simulink model "SELMOTOR_PELICAN_2025"  (R2025b)
settings: Solver=VariableStepAuto  StartTime=0.0  StopTime=5  RelTol=1e-3
settings Model: Creator=juanduque  LastModifiedBy=alvaro
settings SolverCC: AlgebraicLoopSolver=TrustRegion
settings DataIOCC: ReturnWorkspaceOutputs=off
settings OptimizationCC: ReuseModelBlockBuffer=off
settings DebuggingCC: UnconnectedInputMsg=warning  UnconnectedOutputMsg=warning  UnconnectedLineMsg=warning  ArithmeticOperatorsInVariantConditions=warning
settings ModelReferenceCC: EnableRefExpFcnMdlSchedulingChecks=on
settings SFSimCC: SimUseLocalCustomCode=off  CustomCodeUndefinedFunction=UseInterfaceOnly
settings RTWCC: RTWUseLocalCustomCode=off  GPUComputeCapability=3.5
settings CodeAppCC: StateflowObjectComments=on

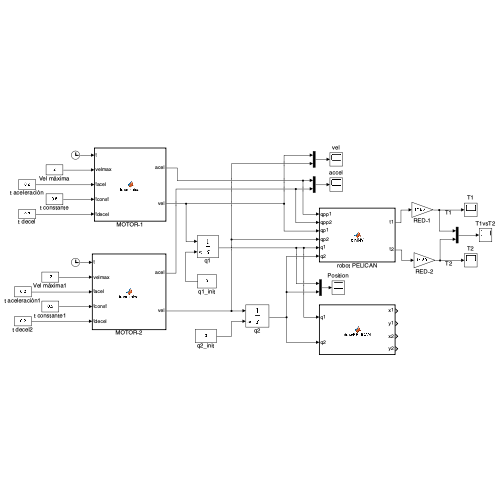
[thumbnail: Simulink's stored preview of the top-level diagram]
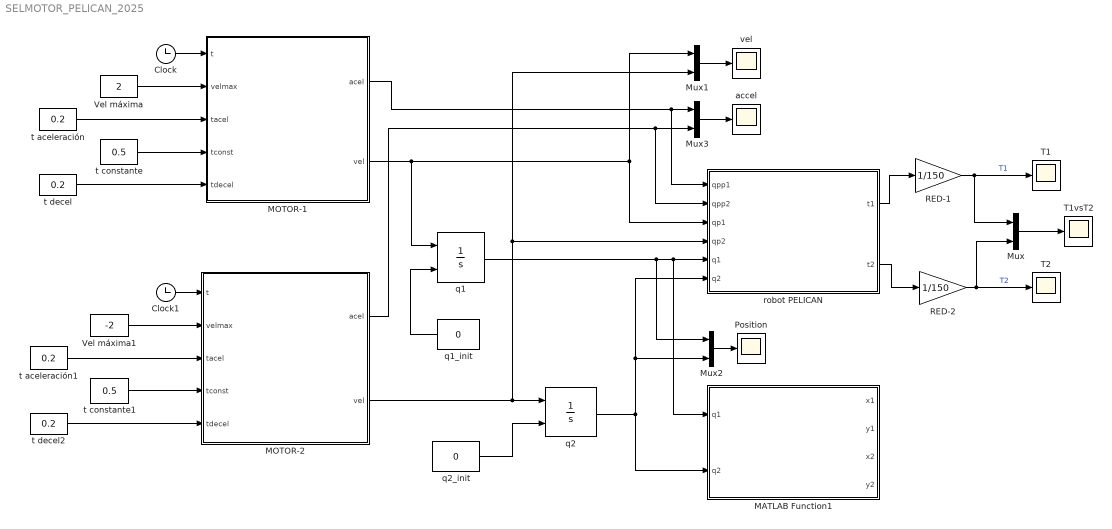
== system SELMOTOR_PELICAN_2025 ==
  Clock : Clock
  Clock1 : Clock
  MATLAB Function1 : MATLAB Function  TreatAsAtomicUnit=on
  MOTOR-1 : MATLAB Function  TreatAsAtomicUnit=on
  MOTOR-2 : MATLAB Function  TreatAsAtomicUnit=on
  Mux{,1..3} (4 alike) : Mux  Inputs=2
  Position : Scope
      settings: ActiveDisplayYMinimum=-1.75  ActiveDisplayYMaximum=1.75  DataLoggingVariableName=ScopeData2
  RED-1 : Gain  Gain=1/150
  RED-2 : Gain  Gain=1/150
  T1 : Scope
      settings: ActiveDisplayYMinimum=0.10997172916761999  ActiveDisplayYMaximum=5.6859934825333962  YLabel=T(t)
  T1vsT2 : Scope
      settings: ActiveDisplayYMinimum=-1.3005259094522184  ActiveDisplayYMaximum=5.8427154423800447  YLabel=T(t)  DataLoggingVariableName=ScopeData3
  T2 : Scope
      settings: ActiveDisplayYMinimum=-1  ActiveDisplayYMaximum=1  YLabel=T(t)  DataLoggingVariableName=ScopeData2
  Vel máxima : Constant  Value=2
  Vel máxima1 : Constant  Value=-2
  accel : Scope
      settings: ActiveDisplayYMinimum=-6.25  ActiveDisplayYMaximum=6.25  DataLoggingVariableName=ScopeData3
  q1 : Integrator  InitialConditionSource=external
  q1_init : Constant  Value=0
  q2 : Integrator  InitialConditionSource=external
  q2_init : Constant  Value=0
  robot PELICAN : MATLAB Function  TreatAsAtomicUnit=on
  t aceleración : Constant  Value=0.2
  t aceleración1 : Constant  Value=0.2
  t constante : Constant  Value=0.5
  t constante1 : Constant  Value=0.5
  t decel : Constant  Value=0.2
  t decel2 : Constant  Value=0.2
  vel : Scope
      settings: ActiveDisplayYMinimum=-1  ActiveDisplayYMaximum=1  YLabel=T(t)
  wires:
  Mux/1 -> T1vsT2/1
  Clock/1 -> MOTOR-1/1(t)
  t decel/1 -> MOTOR-1/5(tdecel)
  t aceleración/1 -> MOTOR-1/3(tacel)
  t constante/1 -> MOTOR-1/4(tconst)
  Vel máxima/1 -> MOTOR-1/2(velmax)
  MOTOR-1/2(vel) -> Mux1/1, robot PELICAN/3(qp1), q1/1
  q1_init/1 -> q1/2
  MOTOR-1/1(acel) -> Mux3/1, robot PELICAN/1(qpp1)
  q2_init/1 -> q2/2
  t aceleración1/1 -> MOTOR-2/3(tacel)
  t constante1/1 -> MOTOR-2/4(tconst)
  MOTOR-2/2(vel) -> q2/1, robot PELICAN/4(qp2), Mux1/2
  t decel2/1 -> MOTOR-2/5(tdecel)
  Clock1/1 -> MOTOR-2/1(t)
  Vel máxima1/1 -> MOTOR-2/2(velmax)
  MOTOR-2/1(acel) -> Mux3/2, robot PELICAN/2(qpp2)
  Mux1/1 -> vel/1
  robot PELICAN/1(t1) -> RED-1/1
  Mux2/1 -> Position/1
  q2/1 -> MATLAB Function1/2(q2), robot PELICAN/6(q2), Mux2/2
  q1/1 -> Mux2/1, robot PELICAN/5(q1), MATLAB Function1/1(q1)
  Mux3/1 -> accel/1
  robot PELICAN/2(t2) -> RED-2/1
  RED-1/1 -> T1/1, Mux/1  "T1"
  RED-2/1 -> T2/1, Mux/2  "T2"

== matlab function SELMOTOR_PELICAN_2025/MOTOR-1 ==
  data: acel output; t input; vel output; velmax input; tacel input; tconst input; tdecel input
% TRAPEZOIDAL  Perfil de velocidad trapezoidal
%    PERFIL=TRAPEZOIDAL(U) devuelve un vector 1x2 que contiene la velocidad 
%    y la aceleración de un perfil de velocidad trapezoidal en un determinado 
%    instante de tiempo. PERFIL(1) contiene la velocidad y PERFIL(2) la 
%    aceleración. U(1) representa el instante de tiempo actual(seg). U(2) es 
%    la velocidad máxima. U(3) es el tiempo de aceleración(seg). U(4) es el
%    tiempo de velocidad constante(seg). U(5) es el tiempo de deceleración(seg).

function [acel, vel]=trapezoidal(t, velmax, tacel, tconst, tdecel)

%t      = u(1);	% Instante de tiempo actual
%velmax = u(2);  % Velocidad máxima
%tacel  = u(3);	% Tiempo de aceleración
% tconst = u(4);	% Tiempo de velocidad constante
% tdecel = u(5);	% Tiempo de deceleración

% Se calcula la velocidad y la aceleración
if t <= tacel
   % Intervalo de aceleración
   acel = velmax/tacel;
   vel  = acel*t;
else
    if t < (tacel+tconst)
	% Intervalo de velocidad constante
        vel  = velmax;
        acel = 0;
    else
        if t>(tacel+tconst+tdecel)
	   % Velocidad y aceleración nula
           vel  = 0;
           acel = 0;
        else
	   % Intervalo de deceleración
           acel = -velmax/tdecel;
           vel  = velmax+acel*(t-tacel-tconst);
        end         
   end
end

% Se devuelve la velocidad y la aceleración
%perfil = [acel vel];

== matlab function SELMOTOR_PELICAN_2025/robot PELICAN ==
  data: qpp1 input; qpp2 input; qp1 input; qp2 input; q1 input; q2 input; t1 output; t2 output
function [t1, t2] = dinINV(qpp1, qpp2, qp1, qp2, q1, q2)


% Parametros del robot
%m1=23.902; m2=3.88;
%L1=0.45; L2=0.45; lc1=0.091;lc2=0.0229;
%I1=1.266; I2=0.093;

% Parametros del robot
m1=33.0; m2=94.4;
L1=0.70; L2=1.02; lc1=0.321;lc2=0.181;
I1=1.57; I2=8.64;

%Matriz de masas
m11= m1*lc1^2 + m2*(L1^2 +lc2^2+2*L1*lc2*cos(q2))+I1+I2;
m12=m2*(lc2^2 +L1*lc2*cos(q2))+I2;
m21=m2*(lc2^2+L1*lc2*cos(q2))+I2
m22=m2*lc2^2+I2;
M=[ m11 m12; m21 m22];
%Matriz de Coriolis
c11=-m2*L1*lc2*sin(q2)*qp2;
c12=-m2*L1*lc2*sin(q2)*(qp1+qp2);
c21=m2*L1*lc2*sin(q2)*qp1;
c22=0;
C=[c11 c12; c21 c22];
%Vector de gravedad
g1=(m1*lc1+m2*L1)*9.8*sin(q1)+m2*lc2*9.8*sin(q1+q2);
g2=m2*lc2*9.8*sin(q1+q2);
G=[g1; g2];
T=M*[qpp1; qpp2]+C*[qp1; qp2]+G;
t1=T(1,1);
t2=T(2,1);

== matlab function SELMOTOR_PELICAN_2025/MOTOR-2 ==
  data: acel output; t input; vel output; velmax input; tacel input; tconst input; tdecel input
% TRAPEZOIDAL  Perfil de velocidad trapezoidal
%    PERFIL=TRAPEZOIDAL(U) devuelve un vector 1x2 que contiene la velocidad 
%    y la aceleración de un perfil de velocidad trapezoidal en un determinado 
%    instante de tiempo. PERFIL(1) contiene la velocidad y PERFIL(2) la 
%    aceleración. U(1) representa el instante de tiempo actual(seg). U(2) es 
%    la velocidad máxima. U(3) es el tiempo de aceleración(seg). U(4) es el
%    tiempo de velocidad constante(seg). U(5) es el tiempo de deceleración(seg).

function [acel, vel]=trapezoidal(t, velmax, tacel, tconst, tdecel)

%t      = u(1);	% Instante de tiempo actual
%velmax = u(2);  % Velocidad máxima
%tacel  = u(3);	% Tiempo de aceleración
% tconst = u(4);	% Tiempo de velocidad constante
% tdecel = u(5);	% Tiempo de deceleración

% Se calcula la velocidad y la aceleración
if t <= tacel
   % Intervalo de aceleración
   acel = velmax/tacel;
   vel  = acel*t;
else
    if t < (tacel+tconst)
	% Intervalo de velocidad constante
        vel  = velmax;
        acel = 0;
    else
        if t>(tacel+tconst+tdecel)
	   % Velocidad y aceleración nula
           vel  = 0;
           acel = 0;
        else
	   % Intervalo de deceleración
           acel = -velmax/tdecel;
           vel  = velmax+acel*(t-tacel-tconst);
        end         
   end
end

% Se devuelve la velocidad y la aceleración
%perfil = [vel acel];

== matlab function SELMOTOR_PELICAN_2025/MATLAB Function1 ==
  data: q1 input; x1 output; q2 input; y1 output; x2 output; y2 output
function [x1,y1,x2,y2] =drawPELICAN(q1, q2)

L1=0.45; L2=0.45;

%	Vector de posicion (x, y, z) de cada sistema de coordenadas
x0 = 0;				    y0 = 0;				
x1 = L1*cos(q1-pi/2);	y1 = L1*sin(q1-pi/2);		
x2 = x1+L2*cos(q1-pi/2+q2);	y2 = y1+L2*sin(q1-pi/2+q2);		

%	Se dibuja el robot
x = [x0 x1 x2];
y = [y0 y1 y2];

plot(x,y);
% Se coloca una rejilla a los ejes
grid;
% Se establecen los límites de los ejes
axis([-1 1 -1 1]);
